simulink library "exampleEnvironment_cl"  (R2018b)
settings: Solver=VariableStepAuto  StartTime=0.0  StopTime=10.0  RelTol=1e-3
settings Model: Creator=mcobb  LastModifiedBy=mcobb

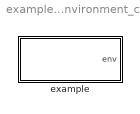
== system exampleEnvironment_cl ==
  example : Subsystem

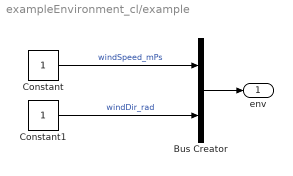
== system exampleEnvironment_cl/example ==
  Bus Creator : BusCreator  Inputs=2
  Constant : Constant
  Constant1 : Constant
  env : Outport  OutDataTypeStr=Bus: envBus
  wires:
  Bus Creator/1 -> env/1
  Constant/1 -> Bus Creator/1  "windSpeed_mPs"
  Constant1/1 -> Bus Creator/2  "windDir_rad"
